simulink model "Bebop_sim_spline_faster"  (R2018a)
settings: Solver=VariableStepAuto  StartTime=0.0  StopTime=100  FixedStep=.05  MaxStep=1  MinStep=0.08  RelTol=1  AbsTol=1
values from neighbouring files (symbols this model uses):
  g = 9.81    [initialize_race_no_realtime.m]    (also in initialize_race_realtime.m; initialize_race_realtime_backup_cubic.m; moving_average_rls_own.m = P(i-1)*meas*(lambda+meas*P(i-1)*meas)^-1)
  max_rot_Z = (90)*pi/180    (= 1.57079632679)    [Bebop_sim_init.m]    (also in initialize_race_no_realtime.m = 1.0471975512; initialize_race_realtime.m; initialize_race_realtime_backup_cubic.m; run_batch1.m = list_agility(idx_agility)*max_rot_Z)
  max_theta_X = (40)*pi/180    (= 0.698131700798)    [Bebop_sim_init.m]    (also in initialize_race_no_realtime.m = 0.13962634016; initialize_race_realtime.m = 1.308996939; initialize_race_realtime_backup_cubic.m = 1.308996939; run_batch1.m = list_agility(idx_agility)*max_theta_X)
  max_theta_Y = (40)*pi/180    (= 0.698131700798)    [Bebop_sim_init.m]    (also in initialize_race_no_realtime.m = 0.13962634016; initialize_race_realtime.m = 1.308996939; initialize_race_realtime_backup_cubic.m = 1.308996939; run_batch1.m = list_agility(idx_agility)*max_theta_Y)
  max_v_Z = .5    (= 0.5)    [Bebop_sim_init.m]    (also in initialize_race_no_realtime.m = 1; initialize_race_realtime.m = 3; initialize_race_realtime_backup_cubic.m = 3; run_batch1.m = list_agility(idx_agility)*max_v_Z)
  splines = zeros(3,4,size(gates,1))    [initialize_race_no_realtime.m]    (also in show_splines.m)
  states_num = size(gates_preflight,1)    [initialize_race_no_realtime.m]    (also in initialize_race_realtime.m = size(flightplan,1); initialize_race_realtime_backup_cubic.m = size(flightplan,1))
undefined symbols (not defined in the file or in its folder): fspecial, gray, Rec, SDTV
libraries: sharedtransform x8, simulink x4, visiontextngfix x2, vrlib x2, aerolibutil x1, visionanalysis x1, visiontransforms x1, visionconversions x1
(part 1 of 2)
settings Model: EnablePacing=on  Creator=vinni  LastModifiedBy=vinni
settings HardwareCC: ProdBitPerLong=64  ProdHWDeviceType=Intel->x86-64 (Linux 64)

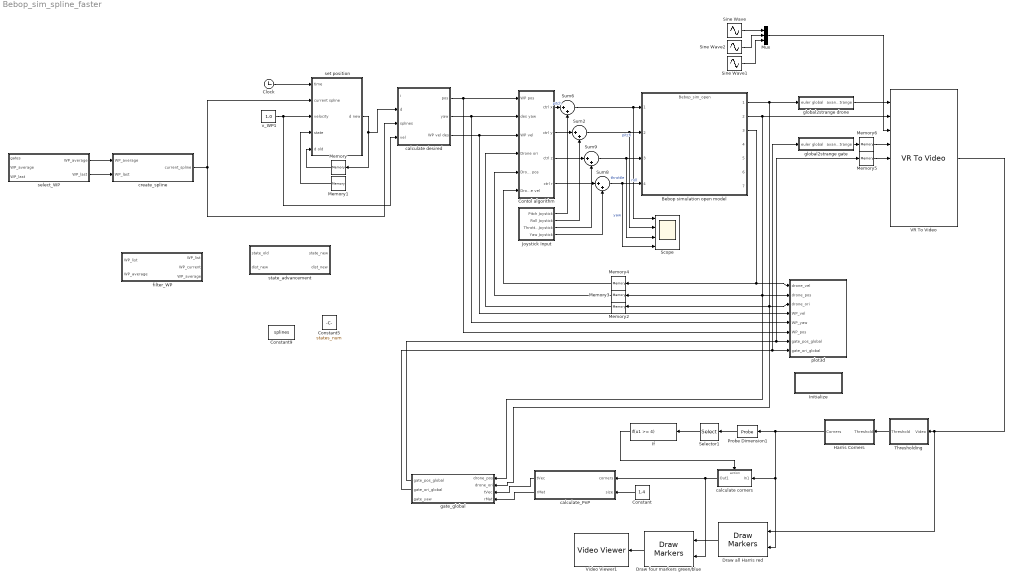
== system Bebop_sim_spline_faster ==
  Bebop simulation open model : ModelReference  ModelNameDialog=Bebop_sim_open.slx  SimulationMode=Normal  ModelReferenceVersion=1.33
  Clock : Clock
  Constant : Constant  Value=1.4
  Constant5 : Constant  Value=states_num
  Constant9 : Constant  Value=splines
  Contol algorithm : Subsystem
  Draw all Harris red : visiontextngfix/Draw Markers  shape=Circle  size=3  fill=on  fillClrSource=Specify via dialog  display=User-specified value  intensity=200  color=[255 0 0]  opacity=1  viewport=Entire image  antialiasing=off  inType=Obsolete  imagePorts=One multidimensional signal  prodOutputMode=Binary point scaling  prodOutputWordLength=32  prodOutputFracLength=14  memoryMode=Specify word length  memoryWordLength=16  memoryFracLength=14  roundingMode=Floor  overflowMode=off
      settings: SourceProductName=Computer Vision System Toolbox  SourceProductBaseCode=VP
  Draw four markers green/blue : visiontextngfix/Draw Markers  shape=Circle  size=3  fill=on  fillClrSource=Specify via dialog  display=User-specified value  intensity=200  color=[0 255 0; 0 0 255;0 0 255; 0 255 0]  opacity=1  viewport=Entire image  antialiasing=off  inType=Obsolete  imagePorts=One multidimensional signal  prodOutputMode=Binary point scaling  prodOutputWordLength=32  prodOutputFracLength=14  memoryMode=Specify word length  memoryWordLength=16  memoryFracLength=14  roundingMode=Floor  overflowMode=off
      settings: SourceProductName=Computer Vision System Toolbox  SourceProductBaseCode=VP
  Harris Corners : Subsystem
  If : If  IfExpression=u1 >= 4  ShowElse=off
  Initialize : Subsystem  TreatAsAtomicUnit=on
  Joystick Input : Subsystem
  Memory{,1..6} (7 alike) : Memory
  Mux : Mux  Inputs=3
  Probe Dimension1 : Probe  ProbeWidth=off  ProbeSampleTime=off  ProbeComplexSignal=off  ProbeSignalDimensions=on
  Scope : Scope  NumInputPorts=4
  Selector1 : Selector  IndexOptions=Index vector (dialog)  Indices=1  OutputSizes=1
  Sine Wave : Sin  Amplitude=0.0  Bias=3  Frequency=0.4  SampleTime=0
  Sine Wave1 : Sin  Amplitude=0.0  Bias=2  Frequency=0.4  SampleTime=0
  Sine Wave2 : Sin  Amplitude=0.0  Frequency=0.4  SampleTime=0
  Sum{2,6,8..9} (4 alike) : Sum  Inputs=|++
  Thresholding : Subsystem
  VR To Video : vrlib/VR To Video  InstantiateOnLoad=on  SampleTime=0.1  ViewEnable=on  RemoteChange=off  RemoteView=off  FieldsWritten=drone.orientation.4.1.1.double#drone.position.3.1.1.double#G1.translation.3.1.1.double#current_gate_red.rotation.4.1.1.double#current_gate_red.translation.3.1.1.double#current_gate_yellow.rotation.4.1.1.double#current_gate_yellow.translation.3.1.1.double#current_gate_green.rotation.4.1.1.double#current_gate_green.translation.3.1.1.double  WorldFileName=race_course.wrl  AutoView=off  VideoDimensions=1*[200 320]  AllowVariableSize=off  FigureProperties="{'Position', 'Name', 'Viewpoint', 'CameraBound', 'CameraDirection', 'CameraPosition', 'CameraUpVector', 'ZoomFactor', 'Antialiasing', 'Headlight', 'Lighting', 'NavPanel', 'Sound', 'StatusBar', 'Stereo3D', 'Stereo3DCameraOffset', 'Stereo3DHIT', 'ToolBar', 'Textures', 'Transparency', 'Triad', 'Wireframe', 'NavZones', 'NavMode', 'NavSpeed', 'CaptureFileFormat', 'CaptureFileName', 'Record2DCompressMethod', 'Record2DCompressQuality', 'Record2D', 'Record2DFileName', 'Record2DFPS'; [3.0000000000000000e+01   6.0000000000000000e+01   3.2000000000000000e+02   2.0000000000000000e+02], '', '_untitled_1', 'on', [0.0000000000000000e+00   0.0000000000000000e+00  -1.0000000000000000e+00], [0.0000000000000000e+00   0.0000000000000000e+00   0.0000000000000000e+00], [0.0000000000000000e+00   1.0000000000000000e+00   0.0000000000000000e+00], [1.0000000000000000e+00], 'on', 'on', 'on', 'none', 'on', 'off', 'off', [1.0000000149011612e-01], [0.0000000000000000e+00], 'off', 'on', 'on', 'none', 'off', 'off', 'fly', 'normal', 'tif', '%f_anim_%n.tif', 'auto', [7.5000000000000000e+01], 'off', '***video***', 'auto'}"
      settings: SourceProductName=Simulink 3D Animation  SourceProductBaseCode=VR
  Video Viewer1 : VideoViewer  colormapValue=gray(256)  FigPos=[828 896 758 735]
  calculate corners : Subsystem  TreatAsAtomicUnit=on
  calculate desired : Subsystem
  calculate_PnP : MATLAB Function  TreatAsAtomicUnit=on
  create_spline : MATLAB Function  TreatAsAtomicUnit=on
  filter_WP : MATLAB Function  TreatAsAtomicUnit=on
  gate_global : MATLAB Function  TreatAsAtomicUnit=on
  global2strange drone : Subsystem
  global2strange gate : Subsystem
  plot3d : MATLAB Function  TreatAsAtomicUnit=on
  select_WP : MATLAB Function  TreatAsAtomicUnit=on
  set position : Subsystem
  state_advancement : MATLAB Function  TreatAsAtomicUnit=on
  v_WP1 : Constant  Value=1.0  VectorParams1D=off
  wires:
  Bebop simulation open model/3 -> Memory4/1, plot3d/1(drone_vel)
  create_spline/1(current_spline) -> calculate desired/3(splines), set position/2(current spline)
  calculate desired/1(pos) -> plot3d/6(WP_pos), Contol algorithm/1(WP pos)
  Clock/1 -> set position/1(time)
  calculate desired/2(yaw) -> plot3d/5(WP_yaw), Contol algorithm/2(des yaw)
  calculate desired/3(WP vel des) -> plot3d/4(WP_vel), Contol algorithm/3(WP vel)
  set position/1(d new) -> Memory/1, calculate desired/2(d)
  Memory/1 -> set position/5(d old)
  Memory1/1 -> set position/4(state)
  v_WP1/1 -> calculate desired/4(vel), set position/3(velocity)
  Memory2/1 -> Contol algorithm/4(Drone ori)
  Memory3/1 -> Contol algorithm/5(Drone pos)
  Memory4/1 -> Contol algorithm/6(Drone vel)
  Sum6/1 -> Scope/1, Bebop simulation open model/1  "pitch"
  Sum2/1 -> Bebop simulation open model/2, Scope/2  "roll"
  Joystick Input/4(Yaw Joystick) -> Sum8/2
  Sum9/1 -> Bebop simulation open model/3, Scope/3  "throttle"
  Joystick Input/2(Roll Joystick) -> Sum2/2
  Joystick Input/1(Pitch Joystick) -> Sum6/2
  Contol algorithm/4(ctrl r) -> Sum8/1
  Contol algorithm/2(ctrl y) -> Sum2/1
  Joystick Input/3(Throttle Joystick) -> Sum9/2
  Contol algorithm/3(ctrl z) -> Sum9/1
  Contol algorithm/1(ctrl x) -> Sum6/1  "pitch"
  Sum8/1 -> Scope/4, Bebop simulation open model/4  "yaw"
  Mux/1 -> VR To Video/3
  Sine Wave1/1 -> Mux/3
  Sine Wave/1 -> Mux/1
  Sine Wave2/1 -> Mux/2
  Bebop simulation open model/2 -> gate_global/1(drone_pos), plot3d/2(drone_pos), Memory3/1, VR To Video/2
  global2strange drone/1(axang strange) -> VR To Video/1
  Draw all Harris red/1 -> Draw four markers green/blue/1
  Probe Dimension1/1 -> Selector1/1
  If/1 -> calculate corners/Action
  VR To Video/1 -> Draw all Harris red/1, Thresholding/1("Video ")
  calculate_PnP/2(rMat) -> gate_global/4(rMat)
  Selector1/1 -> If/1
  calculate_PnP/1(tVec) -> gate_global/3(tVec)
  calculate corners/1(Out1) -> calculate_PnP/1(corners), Draw four markers green/blue/2
  Constant/1 -> calculate_PnP/2(size)
  Draw four markers green/blue/1 -> Video Viewer1/1
  Bebop simulation open model/1 -> Memory2/1, gate_global/2(drone_ori), plot3d/3(drone_ori), global2strange drone/1(euler global)
  Thresholding/1(Threshold) -> Harris Corners/1(Threshold)
  Harris Corners/1(Corners) -> Probe Dimension1/1, Draw all Harris red/2, calculate corners/1(In1)
  gate_global/1(gate_pos_global) -> Memory5/1, plot3d/7(gate_pos_global)
  Memory5/1 -> VR To Video/5
  gate_global/2(gate_ori_global) -> global2strange gate/1(euler global), plot3d/8(gate_ori_global)
  global2strange gate/1(axang strange) -> Memory6/1
  Memory6/1 -> VR To Video/4
  select_WP/1(WP_average) -> create_spline/1(WP_average)
  select_WP/2(WP_last) -> create_spline/2(WP_last)

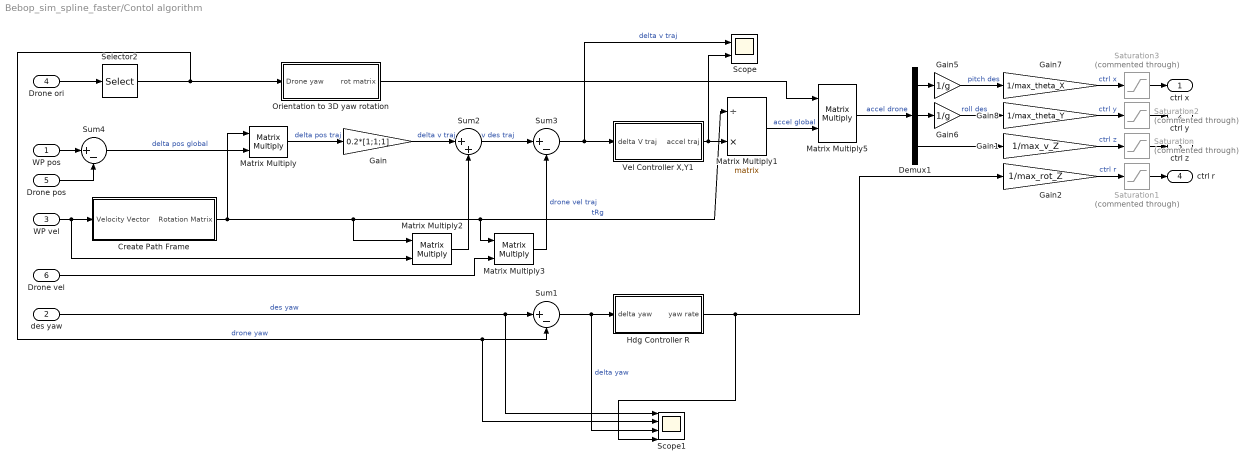
== system Bebop_sim_spline_faster/Contol algorithm ==
  WP pos : Inport
  des yaw : Inport  Port=2
  WP vel : Inport  Port=3
  Drone ori : Inport  Port=4
  Drone pos : Inport  Port=5
  Drone vel : Inport  Port=6
  Create Path Frame : Subsystem
  Demux1 : Demux  Outputs=3
  Gain : Gain  Gain=0.2*[1;1;1]
  Gain1 : Gain  Gain=1/max_v_Z
  Gain2 : Gain  Gain=1/max_rot_Z
  Gain5 : Gain  Gain=1/g
  Gain6 : Gain  Gain=1/g
  Gain7 : Gain  Gain=1/max_theta_X
  Gain8 : Gain  Gain=1/max_theta_Y
  Hdg Controller R : Subsystem
  Matrix Multiply{,2..3,5} (4 alike) : Product  Inputs=**  Multiplication=Matrix(*)
  Matrix Multiply1 : Product  Inputs=/*  Multiplication=Matrix(*)
  Orientation to 3D yaw rotation : Subsystem
  Saturation{,1..3} (4 alike) : Saturate  Commented=through  UpperLimit=1  LowerLimit=-1
  Scope : Scope  NumInputPorts=2
  Scope1 : Scope  NumInputPorts=4
  Selector2 : Selector  InputPortWidth=3  IndexOptions=Index vector (dialog)  Indices=3  OutputSizes=1
  Sum1 : Sum  Inputs=|+-
  Sum2 : Sum  Inputs=|++
  Sum3 : Sum  Inputs=|+-
  Sum4 : Sum  Inputs=|+-
  Vel Controller X,Y1 : Subsystem
  ctrl x : Outport
  ctrl y : Outport  Port=2
  ctrl z : Outport  Port=3
  ctrl r : Outport  Port=4
  wires:
  Sum4/1 -> Matrix Multiply/2  "delta pos global"
  Matrix Multiply/1 -> Gain/1  "delta pos traj"
  Create Path Frame/1(Rotation Matrix) -> Matrix Multiply/1, Matrix Multiply2/1, Matrix Multiply1/1, Matrix Multiply3/1  "tRg"
  WP vel/1 -> Matrix Multiply2/2, Create Path Frame/1(Velocity Vector)
  Drone pos/1 -> Sum4/2
  WP pos/1 -> Sum4/1
  Drone vel/1 -> Matrix Multiply3/2
  Gain/1 -> Sum2/1  "delta v traj"
  Drone ori/1 -> Selector2/1
  des yaw/1 -> Scope1/1, Sum1/1  "des yaw"
  Selector2/1 -> Scope1/2, Sum1/2, Orientation to 3D yaw rotation/1(Drone yaw)  "drone yaw"
  Sum1/1 -> Scope1/3, Hdg Controller R/1(delta yaw)  "delta yaw"
  Hdg Controller R/1(yaw rate) -> Scope1/4, Gain2/1
  Sum2/1 -> Sum3/1  "v des traj"
  Matrix Multiply2/1 -> Sum2/2
  Matrix Multiply3/1 -> Sum3/2  "drone vel traj"
  Sum3/1 -> Scope/1, Vel Controller X,Y1/1(delta V traj)  "delta v traj"
  Matrix Multiply1/1 -> Matrix Multiply5/2  "accel global"
  Vel Controller X,Y1/1(accel traj) -> Scope/2, Matrix Multiply1/2
  Orientation to 3D yaw rotation/1(rot matrix) -> Matrix Multiply5/1
  Matrix Multiply5/1 -> Demux1/1  "accel drone"
  Demux1/1 -> Gain5/1
  Demux1/2 -> Gain6/1
  Gain7/1 -> Saturation3/1  "ctrl x"
  Gain8/1 -> Saturation2/1  "ctrl y"
  Saturation2/1 -> ctrl y/1
  Gain5/1 -> Gain7/1  "pitch des"
  Gain6/1 -> Gain8/1  "roll des"
  Saturation3/1 -> ctrl x/1
  Gain1/1 -> Saturation/1  "ctrl z"
  Saturation/1 -> ctrl z/1
  Demux1/3 -> Gain1/1
  Gain2/1 -> Saturation1/1  "ctrl r"
  Saturation1/1 -> ctrl r/1

== system Bebop_sim_spline_faster/Harris Corners ==
  Threshold : Inport
  Cast To Double : DataTypeConversion  OutDataTypeStr=double
  Corner Detection : visionanalysis/Corner Detection  method=Harris corner detection (Harris & Stephens)  factor=0.01  filter=fspecial('gaussian', [1 9], 3)  thrInten=0.1  thrAngle=157.5  output=Obsolete9b  outputInUse=Corner location  maxNum=5  thrMetric=0.01  neighborSize=[25 25]  isOutVarDim=on  accumMode=Binary point scaling  accumWordLength=32  accumFracLength=0  prodOutputMode=Binary point scaling  prodOutputWordLength=32  prodOutputFracLength=0  memoryMode=Binary point scaling  memoryWordLength=32  memoryFracLength=0  firstCoeffMode=Specify word length  firstCoeffWordLength=16  firstCoeffFracLength=17  roundingMode=Floor  overflowMode=off
      settings: SourceProductName=Computer Vision System Toolbox  SourceProductBaseCode=VP
  Gaussian Pyramid : visiontransforms/Gaussian Pyramid  Commented=on  operation=Expand  level=1  source=Specify via dialog  a=0.375  coef=fspecial('gaussian', [1 9], 3)  hiddenCoef=fspecial('gaussian', [1 9], 3)  firstCoeffMode=Specify word length  firstCoeffWordLength=16  firstCoeffFracLength=17  outputMode=Binary point scaling  outputWordLength=32  outputFracLength=10  prodOutputMode=Binary point scaling  prodOutputWordLength=32  prodOutputFracLength=10  roundingMode=Floor  overflowMode=off
      settings: SourceProductName=Computer Vision System Toolbox  SourceProductBaseCode=VP
  Video Viewer2 : VideoViewer  Commented=on  colormapValue=gray(256)  FigPos=[66 898 768 793]
  Corners : Outport
  wires:
  Threshold/1 -> Cast To Double/1
  Cast To Double/1 -> Gaussian Pyramid/1, Corner Detection/1
  Gaussian Pyramid/1 -> Video Viewer2/1
  Corner Detection/1 -> Corners/1

== system Bebop_sim_spline_faster/Initialize ==
  Event Listener : EventListener  DisableCoverage=on  EventName=reset
  reset_plot : MATLAB Function  TreatAsAtomicUnit=on

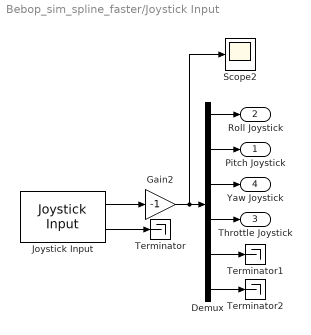
== system Bebop_sim_spline_faster/Joystick Input ==
  Demux : Demux  Outputs=6
  Gain2 : Gain  Gain=-1
  Joystick Input : vrlib/Joystick Input  joyid=1  adjustports=on  forcefeed=off
      settings: SourceProductBaseCode=VR
  Scope2 : Scope
  Terminator : Terminator
  Terminator1 : Terminator
  Terminator2 : Terminator
  Pitch Joystick : Outport
  Roll Joystick : Outport  Port=2
  Throttle Joystick : Outport  Port=3
  Yaw Joystick : Outport  Port=4
  wires:
  Demux/6 -> Terminator2/1
  Demux/5 -> Terminator1/1
  Demux/2 -> Pitch Joystick/1
  Joystick Input/1 -> Gain2/1
  Demux/1 -> Roll Joystick/1
  Demux/3 -> Yaw Joystick/1
  Gain2/1 -> Scope2/1, Demux/1
  Demux/4 -> Throttle Joystick/1
  Joystick Input/2 -> Terminator/1

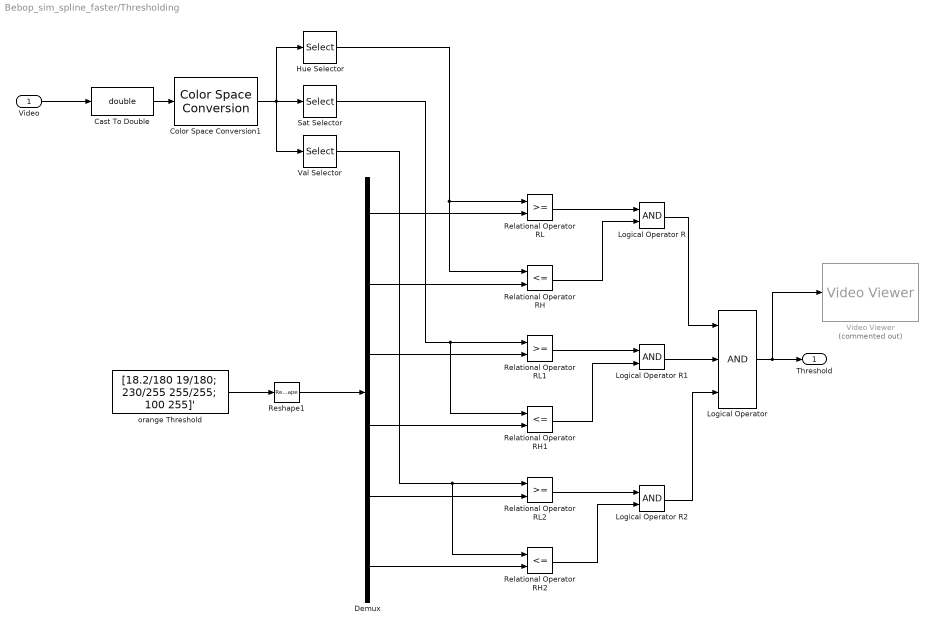
== system Bebop_sim_spline_faster/Thresholding ==
  "Video " : Inport
  Cast To Double : DataTypeConversion  OutDataTypeStr=double
  Color Space Conversion1 : visionconversions/Color Space  Conversion  conversion=Obsolete  conversionActive=R'G'B' to HSV  wp_str=D65  rec=Rec. 601 (SDTV)  sys=1125/60/2:1  imagePorts=One multidimensional signal
      settings: SourceProductName=Computer Vision System Toolbox
  Demux : Demux  Outputs=6
  Hue Selector : Selector  NumberOfDimensions=3  InputPortWidth=3  IndexOptions=Select all,Select all,Index vector (dialog)  Indices=[1 3],1,1  OutputSizes=1,1,1
  Logical Operator : Logic  Inputs=3  AllPortsSameDT=off  OutDataTypeStr=boolean
  Logical Operator R : Logic  AllPortsSameDT=off  OutDataTypeStr=boolean
  Logical Operator R1 : Logic  AllPortsSameDT=off  OutDataTypeStr=boolean
  Logical Operator R2 : Logic  AllPortsSameDT=off  OutDataTypeStr=boolean
  Relational Operator RH : RelationalOperator  Operator=<=  OutDataTypeStr=boolean  RndMeth=Nearest
  Relational Operator RH1 : RelationalOperator  Operator=<=  OutDataTypeStr=boolean  RndMeth=Nearest
  Relational Operator RH2 : RelationalOperator  Operator=<=  OutDataTypeStr=boolean  RndMeth=Nearest
  Relational Operator RL : RelationalOperator  OutDataTypeStr=boolean  RndMeth=Nearest
  Relational Operator RL1 : RelationalOperator  OutDataTypeStr=boolean  RndMeth=Nearest
  Relational Operator RL2 : RelationalOperator  OutDataTypeStr=boolean  RndMeth=Nearest
  Reshape1 : Reshape
  Sat Selector : Selector  NumberOfDimensions=3  InputPortWidth=3  IndexOptions=Select all,Select all,Index vector (dialog)  Indices=[1 3],1,2  OutputSizes=1,1,1
  Val Selector : Selector  NumberOfDimensions=3  InputPortWidth=3  IndexOptions=Select all,Select all,Index vector (dialog)  Indices=[1 3],1,3  OutputSizes=1,1,1
  Video Viewer : VideoViewer  Commented=on  colormapValue=gray(256)  FigPos=[66 898 1535 821]
  orange Threshold : Constant  Value=[18.2/180 19/180; 230/255 255/255; 100 255]'  OutDataTypeStr=double
  Threshold : Outport
  wires:
  Color Space Conversion1/1 -> Val Selector/1, Sat Selector/1, Hue Selector/1
  Demux/6 -> Relational Operator RH2/2
  Val Selector/1 -> Relational Operator RH2/1, Relational Operator RL2/1
  Demux/3 -> Relational Operator RL1/2
  Relational Operator RL/1 -> Logical Operator R/1
  Demux/2 -> Relational Operator RH/2
  orange Threshold/1 -> Reshape1/1
  Cast To Double/1 -> Color Space Conversion1/1
  Demux/5 -> Relational Operator RL2/2
  Hue Selector/1 -> Relational Operator RH/1, Relational Operator RL/1
  Logical Operator R/1 -> Logical Operator/1
  Relational Operator RH/1 -> Logical Operator R/2
  Demux/1 -> Relational Operator RL/2
  Demux/4 -> Relational Operator RH1/2
  "Video "/1 -> Cast To Double/1
  Reshape1/1 -> Demux/1
  Logical Operator R1/1 -> Logical Operator/2
  Relational Operator RH1/1 -> Logical Operator R1/2
  Sat Selector/1 -> Relational Operator RH1/1, Relational Operator RL1/1
  Relational Operator RL1/1 -> Logical Operator R1/1
  Relational Operator RH2/1 -> Logical Operator R2/2
  Relational Operator RL2/1 -> Logical Operator R2/1
  Logical Operator R2/1 -> Logical Operator/3
  Logical Operator/1 -> Video Viewer/1, Threshold/1

== system Bebop_sim_spline_faster/calculate corners ==
  In1 : Inport
  Action Port : ActionPort  PropagateVarSize=During execution  ActionType=then
  MATLAB Function2 : MATLAB Function  TreatAsAtomicUnit=on
  Out1 : Outport
  wires:
  In1/1 -> MATLAB Function2/1(corners)
  MATLAB Function2/1(corners_four) -> Out1/1

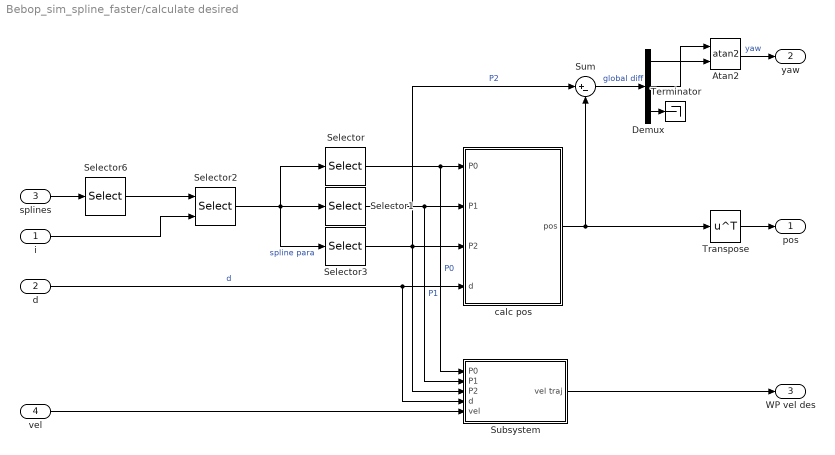
== system Bebop_sim_spline_faster/calculate desired ==
  i : Inport
  d : Inport  Port=2
  splines : Inport  Port=3
  vel : Inport  Port=4
  Atan2 : Trigonometry  Operator=atan2
  Demux : Demux  Outputs=3
  Selector : Selector  NumberOfDimensions=2  InputPortWidth=3  IndexOptions=Index vector (dialog),Select all  Indices=1,1  OutputSizes=1,1
  Selector1 : Selector  NumberOfDimensions=2  InputPortWidth=3  IndexOptions=Index vector (dialog),Select all  Indices=2,1  OutputSizes=1,1
  Selector2 : Selector  NumberOfDimensions=3  IndexMode=Zero-based  InputPortWidth=3  IndexOptions=Select all,Select all,Index vector (port)  Indices=3,1,1  OutputSizes=1,1,1
  Selector3 : Selector  NumberOfDimensions=2  InputPortWidth=3  IndexOptions=Index vector (dialog),Select all  Indices=3,1  OutputSizes=1,1
  Selector6 : Selector  NumberOfDimensions=3  InputPortWidth=3  IndexOptions=Select all,Index vector (dialog),Select all  Indices=3,[1,2,3],1  OutputSizes=1,1,1
  Subsystem : Subsystem
  Sum : Sum  Inputs=|+-
  Terminator : Terminator
  Transpose : Math  Operator=transpose  SaturateOnIntegerOverflow=on
  calc pos : Subsystem
  pos : Outport
  yaw : Outport  Port=2
  WP vel des : Outport  Port=3
  wires:
  splines/1 -> Selector6/1
  i/1 -> Selector2/2
  Selector2/1 -> Selector3/1, Selector1/1, Selector/1  "spline para"
  Selector/1 -> Subsystem/1(P0), calc pos/1(P0)  "P0"
  Selector1/1 -> Subsystem/2(P1), calc pos/2(P1)  "P1"
  Selector3/1 -> Sum/1, Subsystem/3(P2), calc pos/3(P2)  "P2"
  d/1 -> calc pos/4(d), Subsystem/4(d)  "d"
  calc pos/1(pos) -> Sum/2, Transpose/1
  Selector6/1 -> Selector2/1
  Sum/1 -> Demux/1  "global diff"
  Demux/2 -> Atan2/1
  Demux/1 -> Atan2/2
  Demux/3 -> Terminator/1
  Atan2/1 -> yaw/1  "yaw"
  vel/1 -> Subsystem/5(vel)
  Subsystem/1(vel traj) -> WP vel des/1
  Transpose/1 -> pos/1

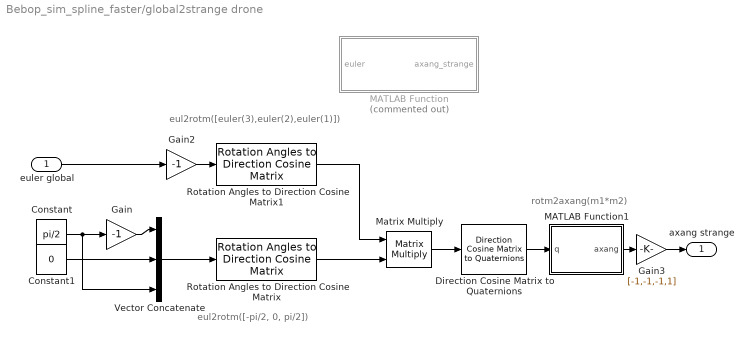
== system Bebop_sim_spline_faster/global2strange drone ==
  note: rotm2axang(m1*m2)
  note: eul2rotm([-pi/2, 0, pi/2])
  note: eul2rotm([euler(3),euler(2),euler(1)])
  euler global : Inport
  Constant : Constant  Value=pi/2
  Constant1 : Constant  Value=0
  Direction Cosine Matrix to Quaternions : sharedtransform/Direction Cosine Matrix  to Quaternions  aMode=0  action=None  tolerance=eps(2)
      settings: SourceProductName=Aerospace Blockset  SourceProductBaseCode=AE
  Gain : Gain  Gain=-1
  Gain2 : Gain  Gain=-1
  Gain3 : Gain  Gain=[-1,-1,-1,1]
  MATLAB Function : MATLAB Function  Commented=on  TreatAsAtomicUnit=on
  MATLAB Function1 : MATLAB Function  TreatAsAtomicUnit=on
  Matrix Multiply : Product  Multiplication=Matrix(*)
  Rotation Angles to Direction Cosine Matrix : sharedtransform/Rotation Angles to Direction Cosine Matrix  rotationOrder=XYZ  aMode=aMode
      settings: SourceProductBaseCode=AE
  Rotation Angles to Direction Cosine Matrix1 : sharedtransform/Rotation Angles to Direction Cosine Matrix  rotationOrder=XYZ  aMode=aMode
      settings: SourceProductBaseCode=AE
  Vector Concatenate : Concatenate  NumInputs=3
  axang strange : Outport
  wires:
  Constant/1 -> Vector Concatenate/3, Gain/1
  Constant1/1 -> Vector Concatenate/2
  Gain/1 -> Vector Concatenate/1
  Rotation Angles to Direction Cosine Matrix/1 -> Matrix Multiply/2
  euler global/1 -> Gain2/1
  Rotation Angles to Direction Cosine Matrix1/1 -> Matrix Multiply/1
  Matrix Multiply/1 -> Direction Cosine Matrix to Quaternions/1
  MATLAB Function1/1(axang) -> Gain3/1
  Vector Concatenate/1 -> Rotation Angles to Direction Cosine Matrix/1
  Gain2/1 -> Rotation Angles to Direction Cosine Matrix1/1
  Direction Cosine Matrix to Quaternions/1 -> MATLAB Function1/1(q)
  Gain3/1 -> axang strange/1

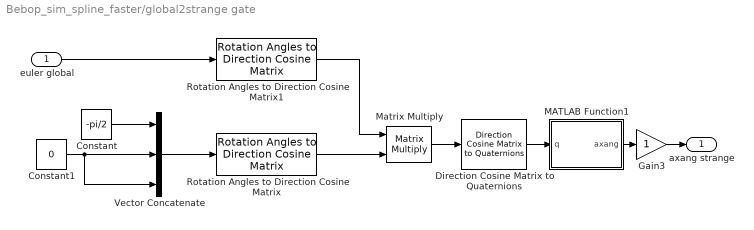
== system Bebop_sim_spline_faster/global2strange gate ==
  euler global : Inport
  Constant : Constant  Value=-pi/2
  Constant1 : Constant  Value=0
  Direction Cosine Matrix to Quaternions : sharedtransform/Direction Cosine Matrix  to Quaternions  aMode=0  action=None  tolerance=eps(2)
      settings: SourceProductName=Aerospace Blockset  SourceProductBaseCode=AE
  Gain3 : Gain
  MATLAB Function1 : MATLAB Function  TreatAsAtomicUnit=on
  Matrix Multiply : Product  Multiplication=Matrix(*)
  Rotation Angles to Direction Cosine Matrix : sharedtransform/Rotation Angles to Direction Cosine Matrix  rotationOrder=ZYX  aMode=aMode
      settings: SourceProductBaseCode=AE
  Rotation Angles to Direction Cosine Matrix1 : sharedtransform/Rotation Angles to Direction Cosine Matrix  rotationOrder=ZYX  aMode=aMode
      settings: SourceProductBaseCode=AE
  Vector Concatenate : Concatenate  NumInputs=3
  axang strange : Outport
  wires:
  Constant/1 -> Vector Concatenate/1
  Rotation Angles to Direction Cosine Matrix/1 -> Matrix Multiply/2
  Rotation Angles to Direction Cosine Matrix1/1 -> Matrix Multiply/1
  Matrix Multiply/1 -> Direction Cosine Matrix to Quaternions/1
  MATLAB Function1/1(axang) -> Gain3/1
  Vector Concatenate/1 -> Rotation Angles to Direction Cosine Matrix/1
  euler global/1 -> Rotation Angles to Direction Cosine Matrix1/1
  Direction Cosine Matrix to Quaternions/1 -> MATLAB Function1/1(q)
  Gain3/1 -> axang strange/1
  Constant1/1 -> Vector Concatenate/3, Vector Concatenate/2

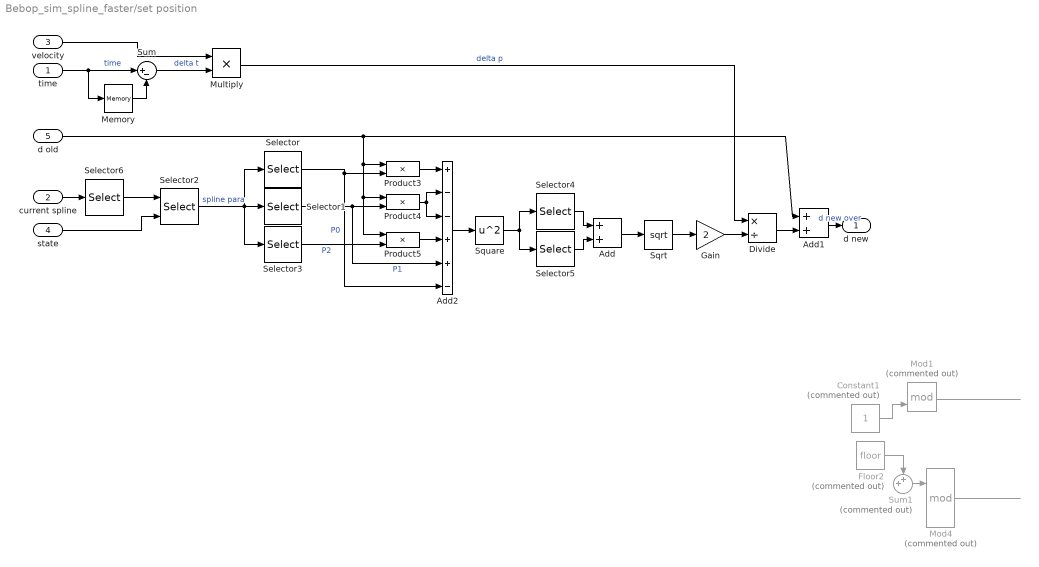
== system Bebop_sim_spline_faster/set position ==
  time : Inport
  current spline : Inport  Port=2
  velocity : Inport  Port=3
  state : Inport  Port=4
  d old : Inport  Port=5
  Add : Sum
  Add1 : Sum
  Add2 : Sum  Inputs=+--++-
  Constant1 : Constant  Commented=on
  Divide : Product  Inputs=*/
  Floor2 : Rounding  Commented=on
  Gain : Gain  Gain=2
  Memory : Memory
  Mod1 : Math  Commented=on  Operator=mod  SaturateOnIntegerOverflow=on
  Mod4 : Math  Commented=on  Operator=mod  SaturateOnIntegerOverflow=on
  Multiply : Product
  Product3 : Product
  Product4 : Product
  Product5 : Product
  Selector : Selector  NumberOfDimensions=2  InputPortWidth=3  IndexOptions=Index vector (dialog),Select all  Indices=1,1  OutputSizes=1,1
  Selector1 : Selector  NumberOfDimensions=2  InputPortWidth=3  IndexOptions=Index vector (dialog),Select all  Indices=2,1  OutputSizes=1,1
  Selector2 : Selector  NumberOfDimensions=3  IndexMode=Zero-based  InputPortWidth=3  IndexOptions=Select all,Select all,Index vector (port)  Indices=3,1,1  OutputSizes=1,1,1
  Selector3 : Selector  NumberOfDimensions=2  InputPortWidth=3  IndexOptions=Index vector (dialog),Select all  Indices=3,1  OutputSizes=1,1
  Selector4 : Selector  InputPortWidth=3  IndexOptions=Index vector (dialog)  Indices=2  OutputSizes=1
  Selector5 : Selector  InputPortWidth=3  IndexOptions=Index vector (dialog)  Indices=1  OutputSizes=1
  Selector6 : Selector  NumberOfDimensions=3  InputPortWidth=3  IndexOptions=Select all,Index vector (dialog),Select all  Indices=3,[1,2,3],1  OutputSizes=1,1,1
  Sqrt : Sqrt  SaturateOnIntegerOverflow=on
  Square : Math  Operator=square  SaturateOnIntegerOverflow=on
  Sum : Sum  Inputs=|+-
  Sum1 : Sum  Commented=on  Inputs=++|
  d new : Outport
  wires:
  time/1 -> Sum/1, Memory/1  "time"
  Memory/1 -> Sum/2
  Sum/1 -> Multiply/2  "delta t"
  velocity/1 -> Multiply/1
  Multiply/1 -> Divide/1  "delta p"
  state/1 -> Selector2/2
  Selector1/1 -> Product4/2, Add2/5  "P1"
  Selector/1 -> Add2/6, Product3/2  "P0"
  current spline/1 -> Selector6/1
  Selector6/1 -> Selector2/1
  Selector2/1 -> Selector/1, Selector3/1, Selector1/1  "spline para"
  Selector5/1 -> Add/2
  d old/1 -> Add1/1, Product5/1, Product4/1, Product3/1
  Add2/1 -> Square/1
  Selector4/1 -> Add/1
  Selector3/1 -> Product5/2  "P2"
  Product4/1 -> Add2/2, Add2/3
  Product3/1 -> Add2/1
  Product5/1 -> Add2/4
  Square/1 -> Selector5/1, Selector4/1
  Add/1 -> Sqrt/1
  Sqrt/1 -> Gain/1
  Gain/1 -> Divide/2
  Divide/1 -> Add1/2
  Add1/1 -> d new/1  "d new over"
  Sum1/1 -> Mod4/1
  ? -> Mod4/2
  Floor2/1 -> Sum1/1
  Mod1/1 -> ?
  Constant1/1 -> Mod1/2
  ? -> Floor2/1  "d new over"
  Mod4/1 -> ?
  ? -> Sum1/2
  ? -> Mod1/1  "d new over"

== system Bebop_sim_spline_faster/Contol algorithm/Create Path Frame ==
  Velocity Vector : Inport
  Invert 3x3 Matrix : aerolibutil/Invert  3x3 Matrix
  Make X Vector : Subsystem
  Make Y Vector : Subsystem
  Make Z Vector : Subsystem
  Matrix Concatenate : Concatenate  NumInputs=3  Mode=Multidimensional array  ConcatenateDimension=2
  Rotation Matrix : Outport
  wires:
  Velocity Vector/1 -> Make Z Vector/1(Velocity Vector), Make X Vector/1(Velocity Vector), Make Y Vector/1(Velocity Vector)
  Make Y Vector/1(Y Vector) -> Matrix Concatenate/2
  Make X Vector/1(X Vector) -> Matrix Concatenate/1
  Make Z Vector/1(Z Vector) -> Matrix Concatenate/3
  Matrix Concatenate/1 -> Invert 3x3 Matrix/1
  Invert 3x3 Matrix/1 -> Rotation Matrix/1

== system Bebop_sim_spline_faster/Contol algorithm/Hdg Controller R ==
  delta yaw : Inport
  Atan2 : Trigonometry  Operator=atan2
  Cos : Trigonometry  Operator=sincos
  PID Controller : simulink/Continuous/PID Controller  Controller=PID  TimeDomain=Continuous-time  SampleTime=-1  IntegratorMethod=Forward Euler  FilterMethod=Forward Euler  Form=Parallel  UseFilter=on  ControllerParametersSource=internal  P=3  I=0.5  D=0  N=10  InitialConditionSource=internal  InitialConditionForIntegrator=0  InitialConditionForFilter=0  ExternalReset=none  LimitOutput=off  UpperSaturationLimit=inf  LowerSaturationLimit=-inf  LinearizeAsGain=on  AntiWindupMode=none  Kb=1  TrackingMode=off  Kt=1  PParamMin=[]  PParamMax=[]  IParamMin=[]  IParamMax=[]  DParamMin=[]  DParamMax=[]  NParamMin=[]  NParamMax=[]  KbParamMin=[]  KbParamMax=[]  KtParamMin=[]  KtParamMax=[]  POutMin=[]  POutMax=[]  IOutMin=[]  IOutMax=[]  DOutMin=[]  DOutMax=[]  NOutMin=[]  NOutMax=[]  KbOutMin=[]  KbOutMax=[]  KtOutMin=[]  KtOutMax=[]  IntegratorOutMin=[]  IntegratorOutMax=[]  FilterOutMin=[]  FilterOutMax=[]  SumOutMin=[]  SumOutMax=[]  SumI1OutMin=[]  SumI1OutMax=[]  SumI2OutMin=[]  SumI2OutMax=[]  SumI3OutMin=[]  SumI3OutMax=[]  SumDOutMin=[]  SumDOutMax=[]  SaturationOutMin=[]  SaturationOutMax=[]  IntegratorContinuousStateAttributes=''  IntegratorStateMustResolveToSignalObject=off  IntegratorRTWStateStorageClass=Auto  FilterContinuousStateAttributes=''  FilterStateMustResolveToSignalObject=off  FilterRTWStateStorageClass=Auto  DifferentiatorICPrevScaledInput=0  DifferentiatorOutMin=[]  DifferentiatorOutMax=[]  FilterDiffOutCoefMin=[]  FilterDiffOutCoefMax=[]  SumDenOutMin=[]  SumDenOutMax=[]  SumNumOutMin=[]  SumNumOutMax=[]  ReciprocalOutMin=[]  ReciprocalOutMax=[]  DivideOutMin=[]  DivideOutMax=[]  TunerSelectOption=Transfer Function Based (PID Tuner App)
  yaw rate : Outport
  wires:
  delta yaw/1 -> Cos/1  "delta yaw"
  Cos/1 -> Atan2/1
  PID Controller/1 -> yaw rate/1  "yaw rate"
  Atan2/1 -> PID Controller/1  "d yaw"
  Cos/2 -> Atan2/2

== system Bebop_sim_spline_faster/Contol algorithm/Orientation to 3D yaw rotation ==
  Drone yaw : Inport
  Constant1 : Constant  Value=0
  Rotation Angles to Direction Cosine Matrix : sharedtransform/Rotation Angles to Direction Cosine Matrix  rotationOrder=ZYX  aMode=aMode
      settings: SourceProductBaseCode=AE
  Vector Concatenate : Concatenate  NumInputs=3
  rot matrix : Outport
  wires:
  Constant1/1 -> Vector Concatenate/2, Vector Concatenate/3
  Vector Concatenate/1 -> Rotation Angles to Direction Cosine Matrix/1
  Drone yaw/1 -> Vector Concatenate/1  "yaw"
  Rotation Angles to Direction Cosine Matrix/1 -> rot matrix/1  "rot matrix"

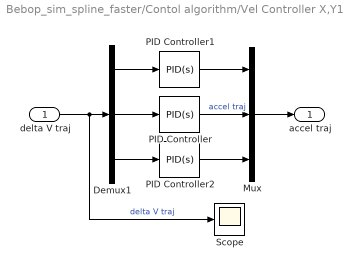
== system Bebop_sim_spline_faster/Contol algorithm/Vel Controller X,Y1 ==
  delta V traj : Inport
  Demux1 : Demux  Outputs=3
  Mux : Mux  Inputs=3
  PID Controller : simulink/Continuous/PID Controller  Controller=PID  TimeDomain=Continuous-time  SampleTime=-1  IntegratorMethod=Forward Euler  FilterMethod=Forward Euler  Form=Parallel  UseFilter=on  ControllerParametersSource=internal  P=4  I=2.5  D=0  N=10  InitialConditionSource=internal  InitialConditionForIntegrator=0  InitialConditionForFilter=0  ExternalReset=none  LimitOutput=off  UpperSaturationLimit=inf  LowerSaturationLimit=-inf  LinearizeAsGain=on  AntiWindupMode=none  Kb=1  TrackingMode=off  Kt=1  PParamMin=[]  PParamMax=[]  IParamMin=[]  IParamMax=[]  DParamMin=[]  DParamMax=[]  NParamMin=[]  NParamMax=[]  KbParamMin=[]  KbParamMax=[]  KtParamMin=[]  KtParamMax=[]  POutMin=[]  POutMax=[]  IOutMin=[]  IOutMax=[]  DOutMin=[]  DOutMax=[]  NOutMin=[]  NOutMax=[]  KbOutMin=[]  KbOutMax=[]  KtOutMin=[]  KtOutMax=[]  IntegratorOutMin=[]  IntegratorOutMax=[]  FilterOutMin=[]  FilterOutMax=[]  SumOutMin=[]  SumOutMax=[]  SumI1OutMin=[]  SumI1OutMax=[]  SumI2OutMin=[]  SumI2OutMax=[]  SumI3OutMin=[]  SumI3OutMax=[]  SumDOutMin=[]  SumDOutMax=[]  SaturationOutMin=[]  SaturationOutMax=[]  IntegratorContinuousStateAttributes=''  IntegratorStateMustResolveToSignalObject=off  IntegratorRTWStateStorageClass=Auto  FilterContinuousStateAttributes=''  FilterStateMustResolveToSignalObject=off  FilterRTWStateStorageClass=Auto  DifferentiatorICPrevScaledInput=0  DifferentiatorOutMin=[]  DifferentiatorOutMax=[]  FilterDiffOutCoefMin=[]  FilterDiffOutCoefMax=[]  SumDenOutMin=[]  SumDenOutMax=[]  SumNumOutMin=[]  SumNumOutMax=[]  ReciprocalOutMin=[]  ReciprocalOutMax=[]  DivideOutMin=[]  DivideOutMax=[]  TunerSelectOption=Transfer Function Based (PID Tuner App)
  PID Controller1 : simulink/Continuous/PID Controller  Controller=PID  TimeDomain=Continuous-time  SampleTime=-1  IntegratorMethod=Forward Euler  FilterMethod=Forward Euler  Form=Parallel  UseFilter=on  ControllerParametersSource=internal  P=4  I=2  D=0  N=10  InitialConditionSource=internal  InitialConditionForIntegrator=0  InitialConditionForFilter=0  ExternalReset=none  LimitOutput=off  UpperSaturationLimit=inf  LowerSaturationLimit=-inf  LinearizeAsGain=on  AntiWindupMode=none  Kb=1  TrackingMode=off  Kt=1  PParamMin=[]  PParamMax=[]  IParamMin=[]  IParamMax=[]  DParamMin=[]  DParamMax=[]  NParamMin=[]  NParamMax=[]  KbParamMin=[]  KbParamMax=[]  KtParamMin=[]  KtParamMax=[]  POutMin=[]  POutMax=[]  IOutMin=[]  IOutMax=[]  DOutMin=[]  DOutMax=[]  NOutMin=[]  NOutMax=[]  KbOutMin=[]  KbOutMax=[]  KtOutMin=[]  KtOutMax=[]  IntegratorOutMin=[]  IntegratorOutMax=[]  FilterOutMin=[]  FilterOutMax=[]  SumOutMin=[]  SumOutMax=[]  SumI1OutMin=[]  SumI1OutMax=[]  SumI2OutMin=[]  SumI2OutMax=[]  SumI3OutMin=[]  SumI3OutMax=[]  SumDOutMin=[]  SumDOutMax=[]  SaturationOutMin=[]  SaturationOutMax=[]  IntegratorContinuousStateAttributes=''  IntegratorStateMustResolveToSignalObject=off  IntegratorRTWStateStorageClass=Auto  FilterContinuousStateAttributes=''  FilterStateMustResolveToSignalObject=off  FilterRTWStateStorageClass=Auto  DifferentiatorICPrevScaledInput=0  DifferentiatorOutMin=[]  DifferentiatorOutMax=[]  FilterDiffOutCoefMin=[]  FilterDiffOutCoefMax=[]  SumDenOutMin=[]  SumDenOutMax=[]  SumNumOutMin=[]  SumNumOutMax=[]  ReciprocalOutMin=[]  ReciprocalOutMax=[]  DivideOutMin=[]  DivideOutMax=[]  TunerSelectOption=Transfer Function Based (PID Tuner App)
  PID Controller2 : simulink/Continuous/PID Controller  Controller=PID  TimeDomain=Continuous-time  SampleTime=-1  IntegratorMethod=Forward Euler  FilterMethod=Forward Euler  Form=Parallel  UseFilter=on  ControllerParametersSource=internal  P=1  I=3  D=0  N=10  InitialConditionSource=internal  InitialConditionForIntegrator=0  InitialConditionForFilter=0  ExternalReset=none  LimitOutput=off  UpperSaturationLimit=inf  LowerSaturationLimit=-inf  LinearizeAsGain=on  AntiWindupMode=none  Kb=1  TrackingMode=off  Kt=1  PParamMin=[]  PParamMax=[]  IParamMin=[]  IParamMax=[]  DParamMin=[]  DParamMax=[]  NParamMin=[]  NParamMax=[]  KbParamMin=[]  KbParamMax=[]  KtParamMin=[]  KtParamMax=[]  POutMin=[]  POutMax=[]  IOutMin=[]  IOutMax=[]  DOutMin=[]  DOutMax=[]  NOutMin=[]  NOutMax=[]  KbOutMin=[]  KbOutMax=[]  KtOutMin=[]  KtOutMax=[]  IntegratorOutMin=[]  IntegratorOutMax=[]  FilterOutMin=[]  FilterOutMax=[]  SumOutMin=[]  SumOutMax=[]  SumI1OutMin=[]  SumI1OutMax=[]  SumI2OutMin=[]  SumI2OutMax=[]  SumI3OutMin=[]  SumI3OutMax=[]  SumDOutMin=[]  SumDOutMax=[]  SaturationOutMin=[]  SaturationOutMax=[]  IntegratorContinuousStateAttributes=''  IntegratorStateMustResolveToSignalObject=off  IntegratorRTWStateStorageClass=Auto  FilterContinuousStateAttributes=''  FilterStateMustResolveToSignalObject=off  FilterRTWStateStorageClass=Auto  DifferentiatorICPrevScaledInput=0  DifferentiatorOutMin=[]  DifferentiatorOutMax=[]  FilterDiffOutCoefMin=[]  FilterDiffOutCoefMax=[]  SumDenOutMin=[]  SumDenOutMax=[]  SumNumOutMin=[]  SumNumOutMax=[]  ReciprocalOutMin=[]  ReciprocalOutMax=[]  DivideOutMin=[]  DivideOutMax=[]  TunerSelectOption=Transfer Function Based (PID Tuner App)
  Scope : Scope
  accel traj : Outport
  wires:
  delta V traj/1 -> Scope/1, Demux1/1  "delta V traj"
  PID Controller/1 -> Mux/2  "accel traj"
  Demux1/1 -> PID Controller1/1
  Demux1/2 -> PID Controller/1
  Demux1/3 -> PID Controller2/1
  PID Controller2/1 -> Mux/3
  PID Controller1/1 -> Mux/1
  Mux/1 -> accel traj/1

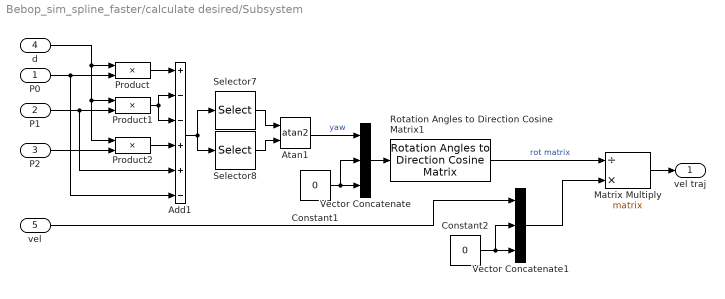
== system Bebop_sim_spline_faster/calculate desired/Subsystem ==
  P0 : Inport
  P1 : Inport  Port=2
  P2 : Inport  Port=3
  d : Inport  Port=4
  vel : Inport  Port=5
  Add1 : Sum  Inputs=+--++-
  Atan1 : Trigonometry  Operator=atan2
  Constant1 : Constant  Value=0
  Constant2 : Constant  Value=0
  Matrix Multiply : Product  Inputs=/*  Multiplication=Matrix(*)
  Product : Product
  Product1 : Product
  Product2 : Product
  Rotation Angles to Direction Cosine Matrix1 : sharedtransform/Rotation Angles to Direction Cosine Matrix  rotationOrder=ZYX  aMode=aMode
      settings: SourceProductBaseCode=AE
  Selector7 : Selector  InputPortWidth=3  IndexOptions=Index vector (dialog)  Indices=2  OutputSizes=1
  Selector8 : Selector  InputPortWidth=3  IndexOptions=Index vector (dialog)  Indices=1  OutputSizes=1
  Vector Concatenate : Concatenate  NumInputs=3
  Vector Concatenate1 : Concatenate  NumInputs=3
  vel traj : Outport
  wires:
  Product2/1 -> Add1/4
  Product1/1 -> Add1/3, Add1/2
  Product/1 -> Add1/1
  Atan1/1 -> Vector Concatenate/1  "yaw"
  Selector7/1 -> Atan1/1
  Constant1/1 -> Vector Concatenate/2, Vector Concatenate/3
  Vector Concatenate1/1 -> Matrix Multiply/2
  P2/1 -> Product2/2
  Matrix Multiply/1 -> vel traj/1
  Vector Concatenate/1 -> Rotation Angles to Direction Cosine Matrix1/1
  P1/1 -> Add1/5, Product1/2
  P0/1 -> Add1/6, Product/2
  d/1 -> Product2/1, Product1/1, Product/1
  Constant2/1 -> Vector Concatenate1/2, Vector Concatenate1/3
  vel/1 -> Vector Concatenate1/1
  Rotation Angles to Direction Cosine Matrix1/1 -> Matrix Multiply/1  "rot matrix"
  Add1/1 -> Selector8/1, Selector7/1
  Selector8/1 -> Atan1/2

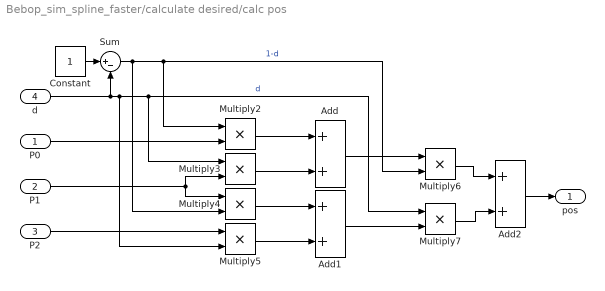
== system Bebop_sim_spline_faster/calculate desired/calc pos ==
  P0 : Inport
  P1 : Inport  Port=2
  P2 : Inport  Port=3
  d : Inport  Port=4
  Add : Sum
  Add1 : Sum
  Add2 : Sum
  Constant : Constant
  Multiply{2..7} (6 alike) : Product
  Sum : Sum  Inputs=|+-
  pos : Outport
  wires:
  d/1 -> Multiply5/2, Multiply7/1, Multiply3/1, Sum/2  "d"
  Sum/1 -> Multiply4/2, Multiply6/2, Multiply2/1  "1-d"
  Constant/1 -> Sum/1
  P0/1 -> Multiply2/2
  P1/1 -> Multiply4/1, Multiply3/2
  P2/1 -> Multiply5/1
  Multiply3/1 -> Add/2
  Multiply2/1 -> Add/1
  Multiply4/1 -> Add1/1
  Multiply5/1 -> Add1/2
  Add/1 -> Multiply6/1
  Add1/1 -> Multiply7/2
  Multiply6/1 -> Add2/1
  Multiply7/1 -> Add2/2
  Add2/1 -> pos/1

== system Bebop_sim_spline_faster/Contol algorithm/Create Path Frame/Make X Vector ==
  Velocity Vector : Inport
  Make Unit : Subsystem
  X Vector : Outport
  wires:
  Velocity Vector/1 -> Make Unit/1(Vector)
  Make Unit/1(Unit Vector) -> X Vector/1

== system Bebop_sim_spline_faster/Contol algorithm/Create Path Frame/Make Y Vector ==
  Velocity Vector : Inport
  Constant : Constant  Value=0
  Demux : Demux  Outputs=3
  Gain : Gain  Gain=-1
  Make Unit : Subsystem
  Matrix Concatenate : Concatenate  NumInputs=3  Mode=Multidimensional array
  Terminator : Terminator
  Y Vector : Outport
  wires:
  Make Unit/1(Unit Vector) -> Y Vector/1
  Velocity Vector/1 -> Demux/1
  Demux/3 -> Terminator/1
  Demux/2 -> Gain/1
  Gain/1 -> Matrix Concatenate/1
  Demux/1 -> Matrix Concatenate/2
  Constant/1 -> Matrix Concatenate/3
  Matrix Concatenate/1 -> Make Unit/1(Vector)

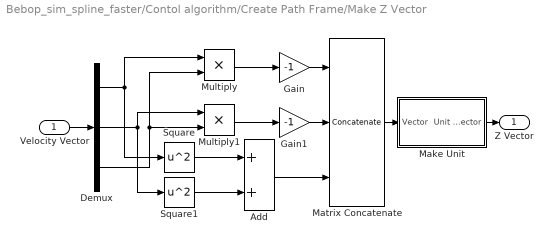
== system Bebop_sim_spline_faster/Contol algorithm/Create Path Frame/Make Z Vector ==
  Velocity Vector : Inport
  Add : Sum
  Demux : Demux  Outputs=3
  Gain : Gain  Gain=-1
  Gain1 : Gain  Gain=-1
  Make Unit : Subsystem
  Matrix Concatenate : Concatenate  NumInputs=3  Mode=Multidimensional array
  Multiply : Product
  Multiply1 : Product
  Square : Math  Operator=square  SaturateOnIntegerOverflow=on
  Square1 : Math  Operator=square  SaturateOnIntegerOverflow=on
  Z Vector : Outport
  wires:
  Make Unit/1(Unit Vector) -> Z Vector/1
  Velocity Vector/1 -> Demux/1
  Demux/3 -> Multiply/2, Multiply1/2
  Matrix Concatenate/1 -> Make Unit/1(Vector)
  Multiply/1 -> Gain/1
  Gain/1 -> Matrix Concatenate/1
  Demux/1 -> Square/1, Multiply/1
  Multiply1/1 -> Gain1/1
  Gain1/1 -> Matrix Concatenate/2
  Demux/2 -> Square1/1, Multiply1/1
  Add/1 -> Matrix Concatenate/3
  Square/1 -> Add/1
  Square1/1 -> Add/2

== system Bebop_sim_spline_faster/Contol algorithm/Create Path Frame/Make X Vector/Make Unit ==
  Vector : Inport
  Multiply : Product
  Reciprocal Sqrt : Sqrt  Operator=rSqrt  SaturateOnIntegerOverflow=on
  Square : Math  Operator=square  SaturateOnIntegerOverflow=on
  Sum of Elements : Sum  Inputs=+
  Unit Vector : Outport
  wires:
  Reciprocal Sqrt/1 -> Multiply/1
  Vector/1 -> Square/1, Multiply/2
  Square/1 -> Sum of Elements/1
  Multiply/1 -> Unit Vector/1
  Sum of Elements/1 -> Reciprocal Sqrt/1

== system Bebop_sim_spline_faster/Contol algorithm/Create Path Frame/Make Y Vector/Make Unit ==
  Vector : Inport
  Multiply : Product
  Reciprocal Sqrt : Sqrt  Operator=rSqrt  SaturateOnIntegerOverflow=on
  Square : Math  Operator=square  SaturateOnIntegerOverflow=on
  Sum of Elements : Sum  Inputs=+
  Unit Vector : Outport
  wires:
  Reciprocal Sqrt/1 -> Multiply/1
  Vector/1 -> Square/1, Multiply/2
  Square/1 -> Sum of Elements/1
  Multiply/1 -> Unit Vector/1
  Sum of Elements/1 -> Reciprocal Sqrt/1

== system Bebop_sim_spline_faster/Contol algorithm/Create Path Frame/Make Z Vector/Make Unit ==
  Vector : Inport
  Multiply : Product
  Reciprocal Sqrt : Sqrt  Operator=rSqrt  SaturateOnIntegerOverflow=on
  Square : Math  Operator=square  SaturateOnIntegerOverflow=on
  Sum of Elements : Sum  Inputs=+
  Unit Vector : Outport
  wires:
  Reciprocal Sqrt/1 -> Multiply/1
  Vector/1 -> Square/1, Multiply/2
  Square/1 -> Sum of Elements/1
  Multiply/1 -> Unit Vector/1
  Sum of Elements/1 -> Reciprocal Sqrt/1

== matlab function Bebop_sim_spline_faster/calculate corners/MATLAB Function2 ==
  data: corners_four output; corners input
function corners_four = calculate_corners(corners)
    
    
    %% get bounding box
    corners = double(corners);
    box=[0,0,0,0];
    box(1) = min(corners(:,1));
    box(2) = max(corners(:,1));
    box(3) = min(corners(:,2));
    box(4) = max(corners(:,2));
    
    corners_box = ([box(1), box(3);
                    box(2), box(3);
                    box(1), box(4);
                    box(2), box(4)]);
                
    corners_four = int32(zeros(4,2));
                
    for m = 1:4
        box = corners_box(m,:);
        multi_box = ones(size(corners,1),1) * box;
        diff = multi_box - corners;
        dist = diff(:,1).^2 + diff(:,2).^2;
        [~,i] = min(dist);
        corners_four(m,:) = corners(i,:);
        corners(i,:)=[];
    end
    
end

== matlab function Bebop_sim_spline_faster/plot3d ==
  data: drone_vel input; drone_pos input; drone_ori input; WP_vel input; WP_yaw input; WP_pos input; gate_pos_global input; gate_ori_global input
function plot3d(drone_vel, drone_pos, drone_ori, WP_vel, WP_yaw, WP_pos, gate_pos_global, gate_ori_global)
coder.extrinsic('delete')

children = get(gca, 'children');
delete(children(1:11));

gRb = eul2rotm([drone_ori(3),drone_ori(2),drone_ori(1)]);
length = 1;
x_bebop = gRb*[length;0;0];
y_bebop = gRb*[0;length;0];
z_bebop = gRb*[0;0;length];


plot3(drone_pos(1),drone_pos(2),drone_pos(3),'m.','MarkerSize',7)
plot3(drone_pos(1),drone_pos(2),0,'k.','MarkerSize',5)

plot3(drone_pos(1)+[0 drone_vel(1)],drone_pos(2)+[0 drone_vel(2)],drone_pos(3)+[0 drone_vel(3)],'k-','LineWidth',2)

plot3(drone_pos(1)+[0 x_bebop(1)],drone_pos(2)+[0 x_bebop(2)],drone_pos(3)+[0 x_bebop(3)],'r-')
plot3(drone_pos(1)+[0 y_bebop(1)],drone_pos(2)+[0 y_bebop(2)],drone_pos(3)+[0 y_bebop(3)],'g-')
plot3(drone_pos(1)+[0 z_bebop(1)],drone_pos(2)+[0 z_bebop(2)],drone_pos(3)+[0 z_bebop(3)],'b-')

plot3(WP_pos(1),WP_pos(2),WP_pos(3),'bx','MarkerSize',10)
plot3(WP_pos(1)+[0 WP_vel(1)],WP_pos(2)+[0 WP_vel(2)],WP_pos(3)+[0 WP_vel(3)],'b-','LineWidth',2)
plot3(WP_pos(1)+[0 cos(WP_yaw)],WP_pos(2)+[0 sin(WP_yaw)],WP_pos(3)+[0 0],'r-','LineWidth',1)


plot3(gate_pos_global(1), gate_pos_global(2), gate_pos_global(3),'ro','LineWidth',2)

gate_rot = eul2rotm(gate_ori_global);
length = 1;
x_gate = gate_rot*[length;0;0];
y_gate = gate_rot*[0;length;0];
z_gate = gate_rot*[0;0;length];
plot3(gate_pos_global(1) + [0 x_gate(1)],gate_pos_global(2) + [0 x_gate(2)],gate_pos_global(3) + [0 x_gate(3)],'r-','LineWidth',2)
plot3(gate_pos_global(1) + [0 y_gate(1)],gate_pos_global(2) + [0 y_gate(2)],gate_pos_global(3) + [0 y_gate(3)],'g-','LineWidth',2)
plot3(gate_pos_global(1) + [0 z_gate(1)],gate_pos_global(2) + [0 z_gate(2)],gate_pos_global(3) + [0 z_gate(3)],'b-','LineWidth',2)

== matlab function Bebop_sim_spline_faster/Initialize/reset_plot ==
function reset_plot()
close all;
figure('units','normalized','outerposition',[0 0 0.5 1])
hold on
grid on
axis equal

for i=1:11
    plot3(0,0,0,'m.')
end

% axis([-5,5,-5,5,-2,2])
axis([-5,5,-5,5,0,4])
%view(-20,40) % 3D view
view(-90,90) % top view
%view(-90,0) % front view
xlabel('x')
ylabel('y')
zlabel('z')

== matlab function Bebop_sim_spline_faster/global2strange drone/MATLAB Function ==
  data: euler input; axang_strange output
function axang_strange = fcn(euler)
m1=zeros(3,3);
m1 = eul2rotm([euler(3),euler(2),euler(1)]);
m2 = eul2rotm([-pi/2, 0, pi/2]);

axang_strange = rotm2axang(m1*m2);

== matlab function Bebop_sim_spline_faster/calculate_PnP ==
  data: tVec output; corners input; size input; rMat output
function [tVec, rMat] = calculate_PnP(corners, size)
    tVec=zeros(1,3);
    rMat=zeros(3,3);
    
    Resolution = 1*[320, 200];
    vertFOV = 1.05;
    f = 0.5*Resolution(2)/tan(0.5*vertFOV);
    IntrinsicMatrix = [f, 0, 0;
        0, f, 0;
        Resolution/2, 1];
    cameraParams = cameraParameters('IntrinsicMatrix',IntrinsicMatrix); 
    
    %% calculate extrinsics
    worldPoints = size/2*[1 1;
        1 -1;
        -1 1;
        -1 -1];
    
    corners=double(corners);
    if corners == zeros(4,2)
        disp('no corners')
        return
    end
    
    angles = zeros(6,1);
    k = 1;
    for m=1:3
        for n=m+1:4
            angles(k)=atan2(corners(m,2)-corners(n,2),corners(m,1)-corners(n,1));
            k = k+1;            
        end
    end
    angles(angles<=0) = angles(angles<=0)+pi;
    
%     a = zeros(2,1);
%     a = hist(angles,unique(angles));
%     if max(a)>2
%         disp('three occurences')
%         return
%     end
%     
%     
%     
    angles = zeros(2,1);
    angles(1)=atan2(corners(1,2)-corners(4,2),corners(1,1)-corners(4,1));
    angles(2)=atan2(corners(2,2)-corners(3,2),corners(2,1)-corners(3,1));
    angles(angles<=0) = angles(angles<=0)+pi;
    
    if ~(isequal(unique(angles),sort(angles)))
        temp = corners(3,:);
        corners(3,:) = corners(4,:);
        corners(4,:) = temp;
    end
    
    angles(1)=atan2(corners(1,2)-corners(4,2),corners(1,1)-corners(4,1));
    angles(2)=atan2(corners(2,2)-corners(3,2),corners(2,1)-corners(3,1));
    angles(angles<=0) = angles(angles<=0)+pi;
    
    if ~(isequal(unique(angles),sort(angles)))
        corners
        disp('still bad after sort')
        return
    end    
    
    [rMat,tVec] = extrinsics(corners,worldPoints,cameraParams);
%     [orientation,location] = extrinsicsToCameraPose(rMat,tVec);
    
end

== matlab function Bebop_sim_spline_faster/gate_global ==
  data: drone_pos input; drone_ori input; gate_pos_global output; tVec input; rMat input; gate_ori_global output; gate_yaw output
function [gate_pos_global, gate_ori_global, gate_yaw]  = gate_global(drone_pos, drone_ori, tVec, rMat)

    gate_pos_global = zeros(3,1);
    gate_ori_global = zeros(1,3);
%     drone_rotm = axang2rotm(drone_ori');
%     gate_pos_local = quatrotate(drone_q,gate_pos_cam);
%     gate_pos_local = drone_rotm * gate_pos_cam';
%     gate_pos_global = gate_pos_local + drone_pos';
%     gate_pos_global = gate_pos_local;
    
    
    %% drone pos
    drone_pos;
    
    
    %% drone orientation
    dRg = eul2rotm([drone_ori(3),drone_ori(2),drone_ori(1)]);
    
    
    %% convert gate pos
    % tVec = right down front, drone was front left up
    dRc = eul2rotm([pi/2,-pi/2,0],'ZYX');
    cRd = dRc^-1;
    cRg = dRg*cRd;
    rel= cRg*tVec';
    gate_pos_global = drone_pos + rel;
    
    % rel = -dRs*tvec';
    % gate_pos_global = drone_pos + rel';
    
    
    %% convert gate orientation
    rot = squeeze(rMat);
    extra = eul2rotm([0,pi/2,0],'ZYX');
    gate_rot = dRg*cRd*rot^-1*extra;
    gate_ori_global = rotm2eul(gate_rot);
%     
%     wRc = rMat;
%     one_more = 1;%eul2rotm([pi,0,-pi/2]);
%     another_one = 1;%eul2rotm([pi/2,0,0]);
%     wRs = another_one*one_more*cRg*wRc;
%     
%     gate_ori_global = (rotm2eul(wRs))';

     gate_yaw = zeros(1,3);
%       rot = rMat*cRg^-1;
%       gate_yaw=rotm2eul(rot);
    
end

== matlab function Bebop_sim_spline_faster/global2strange drone/MATLAB Function1 ==
  data: axang output; q input
function axang = fcn(q)

axang = zeros(4,1);

angle = 2 * acos(q(1));
x = q(2) / sqrt(1-q(1)*q(1));
y = q(3) / sqrt(1-q(1)*q(1));
z = q(4) / sqrt(1-q(1)*q(1));

axang(1) = x;
axang(2) = y;
axang(3) = z;
axang(4) = angle;

== matlab function Bebop_sim_spline_faster/global2strange gate/MATLAB Function1 ==
  data: axang output; q input
function axang = fcn(q)

axang = zeros(4,1);

angle = 2 * acos(q(1));
x = q(2) / sqrt(1-q(1)*q(1));
y = q(3) / sqrt(1-q(1)*q(1));
z = q(4) / sqrt(1-q(1)*q(1));

axang(1) = x;
axang(2) = y;
axang(3) = z;
axang(4) = angle;
